simulink model "Lab_1"  (R2021b)
settings: Solver=ode4  StartTime=0.0  StopTime=10.0  FixedStep=ts  RelTol=1e-3  EnableMultiTasking=on
values from neighbouring files (symbols this model uses):
  ts = 0.01    [matlab.mat]
libraries: arduinolib x1
settings Model: ExtModeTrigDuration=2  Creator=tsuga  LastModifiedBy=karteek
settings SolverCC: AutoInsertRateTranBlk=on
settings DataIOCC: SaveOutput=off  SignalLogging=off  DSMLogging=off  SaveTime=off  ReturnWorkspaceOutputs=off
settings OptimizationCC: DefaultParameterBehavior=Inlined  StrengthReduction=on  PassReuseOutputArgsAs=Individual arguments  ZeroExternalMemoryAtStartup=off  ZeroInternalMemoryAtStartup=off  MaxStackSize=64  OptimizeBlockOrder=speed  OptimizationPriority=Speed  OptimizationCustomize=off  MultiThreadedLoops=on  EfficientTunableParamExpr=on
settings DebuggingCC: ParameterTunabilityLossMsg=error
settings HardwareCC: ProdBitPerInt=16  ProdBitPerPointer=16  ProdBitPerSizeT=16  ProdBitPerPtrDiffT=16  ProdLargestAtomicFloat=None  ProdWordSize=8  ProdHWDeviceType=Atmel->AVR
settings SFSimCC: MATLABDynamicMemAlloc=off
settings RTWCC: Description=Embedded Coder  SystemTargetFile=ert.tlc  HardwareBoard=Arduino Leonardo  TemplateMakefile=ert_default_tmf  Toolchain=Arduino AVR  BuildConfiguration=Faster Runs
settings CodeAppCC: ForceParamTrailComments=on  IgnoreCustomStorageClasses=off  OperatorAnnotations=on  SimulinkDataObjDesc=on  SFDataObjDesc=on  InsertBlockDesc=on
settings ERTTargetCC: SupportContinuousTime=on  SupportVariableSizeSignals=on  ExtModeTransport=5  ExtModeStaticAllocSize=250  ExtModeMexFile=ext_serial_win32_comm_leonardo  InlinedParameterPlacement=NonHierarchical

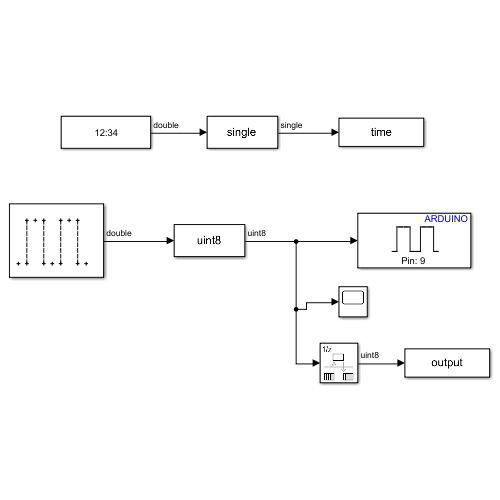
[thumbnail: Simulink's stored preview of the top-level diagram]
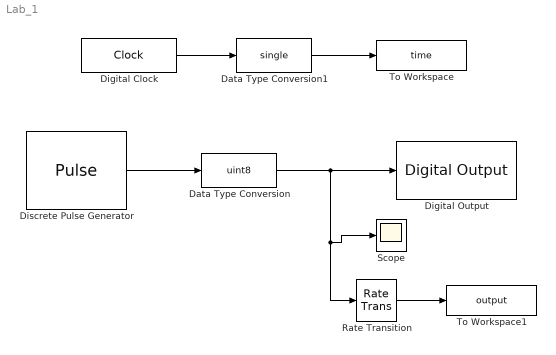
== system Lab_1 ==
  Data Type Conversion : DataTypeConversion  OutDataTypeStr=uint8
  Data Type Conversion1 : DataTypeConversion  OutDataTypeStr=single
  Digital Clock : DigitalClock  SampleTime=ts
  Digital Output : arduinolib/Digital Output  pinNumber=9  Direction=output  blockPlatform=arduino
  Discrete Pulse Generator : DiscretePulseGenerator  Period=10  PulseWidth=2  SampleTime=0.1
  Rate Transition : RateTransition  OutPortSampleTime=ts
  Scope : Scope
  To Workspace : ToWorkspace  VariableName=time  SampleTime=ts
      settings: Save2DSignal=2-D array (concatenate along first dimension)
  To Workspace1 : ToWorkspace  VariableName=output  SampleTime=ts
      settings: Save2DSignal=2-D array (concatenate along first dimension)
  wires:
  Digital Clock/1 -> Data Type Conversion1/1
  Discrete Pulse Generator/1 -> Data Type Conversion/1
  Data Type Conversion/1 -> Scope/1, Rate Transition/1, Digital Output/1
  Data Type Conversion1/1 -> To Workspace/1
  Rate Transition/1 -> To Workspace1/1
